simulink model "RobotArm"  (R2017b)
settings: Solver=FixedStepAuto  StartTime=0.0  StopTime=10  FixedStep=0.01  RelTol=1e-3
values from neighbouring files (symbols this model uses):
  K1 = 0.3415    [PDFUZZY.mat]    (also in gaPI_Fuzzy.m = par(bestchrom,1))
  K2 = 233.0301    [PDFUZZY.mat]    (also in gaPI_Fuzzy.m = par(bestchrom,2))
  K3 = 0.4831    [PDFUZZY.mat]    (also in gaPI_Fuzzy.m = par(bestchrom,3))
  K4 = 261.7584    [PDFUZZY.mat]    (also in gaPI_Fuzzy.m = par(bestchrom,4))
  Kd1 = par(bestchrom,3)-500    [GAthH.m]    (also in PIDVng.mat = 50.32; PIDsine.mat = 47.59; ga.m = par(bestchrom,3))
  Kd2 = par(bestchrom,6)-500    [GAthH.m]    (also in PIDVng.mat = 456.78; PIDsine.mat = 195.5; ga.m = par(bestchrom,6))
  Ki1 = par(bestchrom,2)-500    [GAthH.m]    (also in PIDVng.mat = 842.19; PIDsine.mat = 22.71; ga.m = par(bestchrom,2))
  Ki2 = par(bestchrom,5)-500    [GAthH.m]    (also in PIDVng.mat = 818.9; PIDsine.mat = 632.08; ga.m = par(bestchrom,5))
  Kp1 = par(bestchrom,1)-500    [GAthH.m]    (also in PIDVng.mat = 37.19; PIDsine.mat = 1.19; ga.m = par(bestchrom,1))
  Kp2 = par(bestchrom,4)-500    [GAthH.m]    (also in PIDVng.mat = 595.8; PIDsine.mat = 711.73; ga.m = par(bestchrom,4))
libraries: neural x50, fuzblock x2
(part 2 of 2)

== system RobotArm/PD_FUZZY_NEURAL /Custom Neural Network/Layer 2/LW{2,1} ==
  "ad{2,1}" : Inport  PortDimensions=20
      mask Display: e = 0.06;c1 = [120 230 180]/255;c2 = ([120 230 180]+0)/(256+128);c3 = ([120 230 180]+128)/(256+128);patch([0 1 1 0],[0 0 1 1],c1);patch([0 1 1 1-e 1-e 0+e],[0 0 1 1-e 0+e 0+e],c2);patch([0 0 1 1-e 0+e 0+e],[0 1 1 1-e 1-e 0+e],c3);plot([0 1 1 0 0],[0 0 1 1 0]);
  "IW{2,1}(1,:)'" : Constant  Value=[0.046554121912123817839113115724103408865630626678466796875;0.00016778847839335527133107495156849608974880538880825042724609375;0.01578686841424471742900692561306641437113285064697265625;-0.239614599437442177265467080360394902527332305908203125;-0.00822580942548027140015509672821281128562986850738525390625;-0.0333527887051501270576636670739389955997467041015625;0.006210181379244878070722268859071846236474812030792236328125;0.00900374076438229149765835046537176822312176227569580078125;-0.69848343780560673277335581587976776063442230224609375;-0.00280046923413862676455199363090287079103291034698486328125;0.004350649853579568841766000986126528005115687847137451171875;0.0662036547980797696055788037483580410480499267578125;0.004075788378211603855960643016942412941716611385345458984375;-0.64280666178294254553549080810626037418842315673828125;-0.0026488012173344521911488858023631109972484409809112548828125;-0.002129328380407683428410248183126896037720143795013427734375;-0.428133034077831264863078786220285110175609588623046875;0.129127304962275035737917505684890784323215484619140625;-0.006878772900469370087106479871863484731875360012054443359375;-0.0248842172997741743756261456610445748083293437957763671875]
      mask Display: e = 0.06;c1 = [120 150 230]/255;c2 = ([120 150 230]+0)/383;c3 = ([120 150 230]+128)/383;patch([0 1 1 0],[0 0 1 1],c1);patch([0 1 1 1-e 1-e 0+e],[0 0 1 1-e 0+e 0+e],c2);patch([0 0 1 1-e 0+e 0+e],[0 1 1 1-e 1-e 0+e],c3);plot([0 1 1 0 0],[0 0 1 1 0]);disp('weights');
  Mux : Mux  Inputs=1
      mask Display: e = 0.06;c1 = [120 150 230]/255;c2 = ([120 150 230]+0)/383;c3 = ([120 150 230]+128)/383;patch([0 1 1 0],[0 0 1 1],c1);patch([0 1 1 1-e 1-e 0+e],[0 0 1 1-e 0+e 0+e],c2);patch([0 0 1 1-e 0+e 0+e],[0 1 1 1-e 1-e 0+e],c3);plot([0 1 1 0 0],[0 0 1 1 0]);disp('Mux');
  dotprod1 : neural/Weight Functions/dotprod
      settings: SourceProductName=MATLAB Runtime - Deep Learning Toolbox  SourceProductBaseCode=Missing
  "lz{2,1}" : Outport
      mask Display: e = 0.06;c1 = [120 230 180]/255;c2 = ([120 230 180]+0)/(256+128);c3 = ([120 230 180]+128)/(256+128);patch([0 1 1 0],[0 0 1 1],c1);patch([0 1 1 1-e 1-e 0+e],[0 0 1 1-e 0+e 0+e],c2);patch([0 0 1 1-e 0+e 0+e],[0 1 1 1-e 1-e 0+e],c3);plot([0 1 1 0 0],[0 0 1 1 0]);
  wires:
  "IW{2,1}(1,:)'"/1 -> dotprod1/1
  "ad{2,1}"/1 -> dotprod1/2
  dotprod1/1 -> Mux/1
  Mux/1 -> "lz{2,1}"/1

== system RobotArm/PD_FUZZY_NEURAL /Custom Neural Network1/Layer 1/Delays 1 ==
  "p{1}" : Inport  PortDimensions=3
      mask Display: e = 0.06;c1 = [120 230 180]/255;c2 = ([120 230 180]+0)/(256+128);c3 = ([120 230 180]+128)/(256+128);patch([0 1 1 0],[0 0 1 1],c1);patch([0 1 1 1-e 1-e 0+e],[0 0 1 1-e 0+e 0+e],c2);patch([0 0 1 1-e 0+e 0+e],[0 1 1 1-e 1-e 0+e],c3);plot([0 1 1 0 0],[0 0 1 1 0]);
  mux : Mux  Inputs=1
      mask Display: e = 0.06;c1 = [120 150 230]/255;c2 = ([120 150 230]+0)/383;c3 = ([120 150 230]+128)/383;patch([0 1 1 0],[0 0 1 1],c1);patch([0 1 1 1-e 1-e 0+e],[0 0 1 1-e 0+e 0+e],c2);patch([0 0 1 1-e 0+e 0+e],[0 1 1 1-e 1-e 0+e],c3);plot([0 1 1 0 0],[0 0 1 1 0]);disp('Mux')
  "pd{1,1}" : Outport
      mask Display: e = 0.06;c1 = [120 230 180]/255;c2 = ([120 230 180]+0)/(256+128);c3 = ([120 230 180]+128)/(256+128);patch([0 1 1 0],[0 0 1 1],c1);patch([0 1 1 1-e 1-e 0+e],[0 0 1 1-e 0+e 0+e],c2);patch([0 0 1 1-e 0+e 0+e],[0 1 1 1-e 1-e 0+e],c3);plot([0 1 1 0 0],[0 0 1 1 0]);
  wires:
  "p{1}"/1 -> mux/1
  mux/1 -> "pd{1,1}"/1

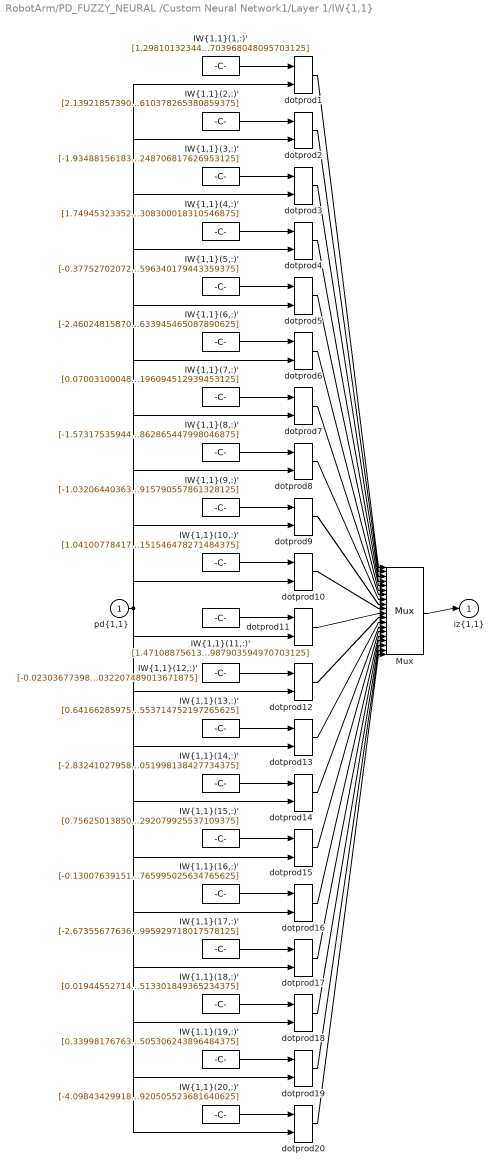
== system RobotArm/PD_FUZZY_NEURAL /Custom Neural Network1/Layer 1/IW{1,1} ==
  "pd{1,1}" : Inport  PortDimensions=3
      mask Display: e = 0.06;c1 = [120 230 180]/255;c2 = ([120 230 180]+0)/(256+128);c3 = ([120 230 180]+128)/(256+128);patch([0 1 1 0],[0 0 1 1],c1);patch([0 1 1 1-e 1-e 0+e],[0 0 1 1-e 0+e 0+e],c2);patch([0 0 1 1-e 0+e 0+e],[0 1 1 1-e 1-e 0+e],c3);plot([0 1 1 0 0],[0 0 1 1 0]);
  "IW{1,1}(1,:)'" : Constant  Value=[1.298101323448510147073875486967153847217559814453125;2.68668995949206479423310156562365591526031494140625;0.105680713798559811067434566211886703968048095703125]
      mask Display: e = 0.06;c1 = [120 150 230]/255;c2 = ([120 150 230]+0)/383;c3 = ([120 150 230]+128)/383;patch([0 1 1 0],[0 0 1 1],c1);patch([0 1 1 1-e 1-e 0+e],[0 0 1 1-e 0+e 0+e],c2);patch([0 0 1 1-e 0+e 0+e],[0 1 1 1-e 1-e 0+e],c3);plot([0 1 1 0 0],[0 0 1 1 0]);disp('Weights');
  "IW{1,1}(10,:)'" : Constant  Value=[1.041007784178143769082680591964162886142730712890625;1.0913679189835960858800945061375387012958526611328125;-3.79403971379421900422812541364692151546478271484375]
      mask Display: e = 0.06;c1 = [120 150 230]/255;c2 = ([120 150 230]+0)/383;c3 = ([120 150 230]+128)/383;patch([0 1 1 0],[0 0 1 1],c1);patch([0 1 1 1-e 1-e 0+e],[0 0 1 1-e 0+e 0+e],c2);patch([0 0 1 1-e 0+e 0+e],[0 1 1 1-e 1-e 0+e],c3);plot([0 1 1 0 0],[0 0 1 1 0]);disp('Weights');
  "IW{1,1}(11,:)'" : Constant  Value=[1.4710887561372587573060854992945678532123565673828125;-2.594021154299451126234998810105025768280029296875;-0.55809622186945173627492522427928633987903594970703125]
      mask Display: e = 0.06;c1 = [120 150 230]/255;c2 = ([120 150 230]+0)/383;c3 = ([120 150 230]+128)/383;patch([0 1 1 0],[0 0 1 1],c1);patch([0 1 1 1-e 1-e 0+e],[0 0 1 1-e 0+e 0+e],c2);patch([0 0 1 1-e 0+e 0+e],[0 1 1 1-e 1-e 0+e],c3);plot([0 1 1 0 0],[0 0 1 1 0]);disp('Weights');
  "IW{1,1}(12,:)'" : Constant  Value=[-0.02303677398099664153097165808503632433712482452392578125;-0.76517648256534098738512739146244712173938751220703125;0.019126199468667948178079996068845503032207489013671875]
      mask Display: e = 0.06;c1 = [120 150 230]/255;c2 = ([120 150 230]+0)/383;c3 = ([120 150 230]+128)/383;patch([0 1 1 0],[0 0 1 1],c1);patch([0 1 1 1-e 1-e 0+e],[0 0 1 1-e 0+e 0+e],c2);patch([0 0 1 1-e 0+e 0+e],[0 1 1 1-e 1-e 0+e],c3);plot([0 1 1 0 0],[0 0 1 1 0]);disp('Weights');
  "IW{1,1}(13,:)'" : Constant  Value=[0.641662859756776615682838382781483232975006103515625;1.648229245395270492480221946607343852519989013671875;3.25430695858256147090514787123538553714752197265625]
      mask Display: e = 0.06;c1 = [120 150 230]/255;c2 = ([120 150 230]+0)/383;c3 = ([120 150 230]+128)/383;patch([0 1 1 0],[0 0 1 1],c1);patch([0 1 1 1-e 1-e 0+e],[0 0 1 1-e 0+e 0+e],c2);patch([0 0 1 1-e 0+e 0+e],[0 1 1 1-e 1-e 0+e],c3);plot([0 1 1 0 0],[0 0 1 1 0]);disp('Weights');
  "IW{1,1}(14,:)'" : Constant  Value=[-2.83241027958725322122290890547446906566619873046875;-2.545638294362128295489355878089554607868194580078125;1.7885263091579071126346889286651276051998138427734375]
      mask Display: e = 0.06;c1 = [120 150 230]/255;c2 = ([120 150 230]+0)/383;c3 = ([120 150 230]+128)/383;patch([0 1 1 0],[0 0 1 1],c1);patch([0 1 1 1-e 1-e 0+e],[0 0 1 1-e 0+e 0+e],c2);patch([0 0 1 1-e 0+e 0+e],[0 1 1 1-e 1-e 0+e],c3);plot([0 1 1 0 0],[0 0 1 1 0]);disp('Weights');
  "IW{1,1}(15,:)'" : Constant  Value=[0.75625013850906885881641983360168524086475372314453125;2.0612501133497556082829760271124541759490966796875;3.430399247565897979939109063707292079925537109375]
      mask Display: e = 0.06;c1 = [120 150 230]/255;c2 = ([120 150 230]+0)/383;c3 = ([120 150 230]+128)/383;patch([0 1 1 0],[0 0 1 1],c1);patch([0 1 1 1-e 1-e 0+e],[0 0 1 1-e 0+e 0+e],c2);patch([0 0 1 1-e 0+e 0+e],[0 1 1 1-e 1-e 0+e],c3);plot([0 1 1 0 0],[0 0 1 1 0]);disp('Weights');
  "IW{1,1}(16,:)'" : Constant  Value=[-0.1300763915144957649783208353255758993327617645263671875;3.1475687752719210266150184907019138336181640625;-0.168673167062670492644116393421427346765995025634765625]
      mask Display: e = 0.06;c1 = [120 150 230]/255;c2 = ([120 150 230]+0)/383;c3 = ([120 150 230]+128)/383;patch([0 1 1 0],[0 0 1 1],c1);patch([0 1 1 1-e 1-e 0+e],[0 0 1 1-e 0+e 0+e],c2);patch([0 0 1 1-e 0+e 0+e],[0 1 1 1-e 1-e 0+e],c3);plot([0 1 1 0 0],[0 0 1 1 0]);disp('Weights');
  "IW{1,1}(17,:)'" : Constant  Value=[-2.673556776367207010736137817730195820331573486328125;-1.71981529092930518487492008716799318790435791015625;-0.450613133605147375693178446454112417995929718017578125]
      mask Display: e = 0.06;c1 = [120 150 230]/255;c2 = ([120 150 230]+0)/383;c3 = ([120 150 230]+128)/383;patch([0 1 1 0],[0 0 1 1],c1);patch([0 1 1 1-e 1-e 0+e],[0 0 1 1-e 0+e 0+e],c2);patch([0 0 1 1-e 0+e 0+e],[0 1 1 1-e 1-e 0+e],c3);plot([0 1 1 0 0],[0 0 1 1 0]);disp('Weights');
  "IW{1,1}(18,:)'" : Constant  Value=[0.019445527148039480624941433006824809126555919647216796875;0.9852408339296356842851309920661151409149169921875;0.02175143784294740478824081719722016714513301849365234375]
      mask Display: e = 0.06;c1 = [120 150 230]/255;c2 = ([120 150 230]+0)/383;c3 = ([120 150 230]+128)/383;patch([0 1 1 0],[0 0 1 1],c1);patch([0 1 1 1-e 1-e 0+e],[0 0 1 1-e 0+e 0+e],c2);patch([0 0 1 1-e 0+e 0+e],[0 1 1 1-e 1-e 0+e],c3);plot([0 1 1 0 0],[0 0 1 1 0]);disp('Weights');
  "IW{1,1}(19,:)'" : Constant  Value=[0.339981767632175746474132438379456289112567901611328125;-3.835244849837684544269222897128202021121978759765625;-1.3542732867112066141856985268532298505306243896484375]
      mask Display: e = 0.06;c1 = [120 150 230]/255;c2 = ([120 150 230]+0)/383;c3 = ([120 150 230]+128)/383;patch([0 1 1 0],[0 0 1 1],c1);patch([0 1 1 1-e 1-e 0+e],[0 0 1 1-e 0+e 0+e],c2);patch([0 0 1 1-e 0+e 0+e],[0 1 1 1-e 1-e 0+e],c3);plot([0 1 1 0 0],[0 0 1 1 0]);disp('Weights');
  "IW{1,1}(2,:)'" : Constant  Value=[2.1392185739000684208122038398869335651397705078125;1.281674728313323186057459679432213306427001953125;3.641787407070763205041430410346947610378265380859375]
      mask Display: e = 0.06;c1 = [120 150 230]/255;c2 = ([120 150 230]+0)/383;c3 = ([120 150 230]+128)/383;patch([0 1 1 0],[0 0 1 1],c1);patch([0 1 1 1-e 1-e 0+e],[0 0 1 1-e 0+e 0+e],c2);patch([0 0 1 1-e 0+e 0+e],[0 1 1 1-e 1-e 0+e],c3);plot([0 1 1 0 0],[0 0 1 1 0]);disp('Weights');
  "IW{1,1}(20,:)'" : Constant  Value=[-4.09843429918166979319948950433172285556793212890625;0.69057330462055477315885809730389155447483062744140625;0.0223408364389678683326057040403611608780920505523681640625]
      mask Display: e = 0.06;c1 = [120 150 230]/255;c2 = ([120 150 230]+0)/383;c3 = ([120 150 230]+128)/383;patch([0 1 1 0],[0 0 1 1],c1);patch([0 1 1 1-e 1-e 0+e],[0 0 1 1-e 0+e 0+e],c2);patch([0 0 1 1-e 0+e 0+e],[0 1 1 1-e 1-e 0+e],c3);plot([0 1 1 0 0],[0 0 1 1 0]);disp('Weights');
  "IW{1,1}(3,:)'" : Constant  Value=[-1.93488156183017512290689410292543470859527587890625;2.103172833789326734432734156143851578235626220703125;-2.540487994611002608991157103446312248706817626953125]
      mask Display: e = 0.06;c1 = [120 150 230]/255;c2 = ([120 150 230]+0)/383;c3 = ([120 150 230]+128)/383;patch([0 1 1 0],[0 0 1 1],c1);patch([0 1 1 1-e 1-e 0+e],[0 0 1 1-e 0+e 0+e],c2);patch([0 0 1 1-e 0+e 0+e],[0 1 1 1-e 1-e 0+e],c3);plot([0 1 1 0 0],[0 0 1 1 0]);disp('Weights');
  "IW{1,1}(4,:)'" : Constant  Value=[1.7494532335268075939893606118857860565185546875;3.050495676388021326630450857919640839099884033203125;-0.92830260598007707795176202125730924308300018310546875]
      mask Display: e = 0.06;c1 = [120 150 230]/255;c2 = ([120 150 230]+0)/383;c3 = ([120 150 230]+128)/383;patch([0 1 1 0],[0 0 1 1],c1);patch([0 1 1 1-e 1-e 0+e],[0 0 1 1-e 0+e 0+e],c2);patch([0 0 1 1-e 0+e 0+e],[0 1 1 1-e 1-e 0+e],c3);plot([0 1 1 0 0],[0 0 1 1 0]);disp('Weights');
  "IW{1,1}(5,:)'" : Constant  Value=[-0.37752702072625432538899303835933096706867218017578125;-1.137271367403070332358083760482259094715118408203125;1.551047187862562903859497964731417596340179443359375]
      mask Display: e = 0.06;c1 = [120 150 230]/255;c2 = ([120 150 230]+0)/383;c3 = ([120 150 230]+128)/383;patch([0 1 1 0],[0 0 1 1],c1);patch([0 1 1 1-e 1-e 0+e],[0 0 1 1-e 0+e 0+e],c2);patch([0 0 1 1-e 0+e 0+e],[0 1 1 1-e 1-e 0+e],c3);plot([0 1 1 0 0],[0 0 1 1 0]);disp('Weights');
  "IW{1,1}(6,:)'" : Constant  Value=[-2.460248158700125031828065402805805206298828125;0.84061468188021704062151684411219321191310882568359375;2.31296954212943006723435246385633945465087890625]
      mask Display: e = 0.06;c1 = [120 150 230]/255;c2 = ([120 150 230]+0)/383;c3 = ([120 150 230]+128)/383;patch([0 1 1 0],[0 0 1 1],c1);patch([0 1 1 1-e 1-e 0+e],[0 0 1 1-e 0+e 0+e],c2);patch([0 0 1 1-e 0+e 0+e],[0 1 1 1-e 1-e 0+e],c3);plot([0 1 1 0 0],[0 0 1 1 0]);disp('Weights');
  "IW{1,1}(7,:)'" : Constant  Value=[0.0700310004863720914070057688149972818791866302490234375;-1.6712400212012938904848624588339589536190032958984375;-0.0815120027134079994102222599394735880196094512939453125]
      mask Display: e = 0.06;c1 = [120 150 230]/255;c2 = ([120 150 230]+0)/383;c3 = ([120 150 230]+128)/383;patch([0 1 1 0],[0 0 1 1],c1);patch([0 1 1 1-e 1-e 0+e],[0 0 1 1-e 0+e 0+e],c2);patch([0 0 1 1-e 0+e 0+e],[0 1 1 1-e 1-e 0+e],c3);plot([0 1 1 0 0],[0 0 1 1 0]);disp('Weights');
  "IW{1,1}(8,:)'" : Constant  Value=[-1.5731753594485500258315369137562811374664306640625;-1.1714016532727262731583550703362561762332916259765625;3.363686937816534605616425324114970862865447998046875]
      mask Display: e = 0.06;c1 = [120 150 230]/255;c2 = ([120 150 230]+0)/383;c3 = ([120 150 230]+128)/383;patch([0 1 1 0],[0 0 1 1],c1);patch([0 1 1 1-e 1-e 0+e],[0 0 1 1-e 0+e 0+e],c2);patch([0 0 1 1-e 0+e 0+e],[0 1 1 1-e 1-e 0+e],c3);plot([0 1 1 0 0],[0 0 1 1 0]);disp('Weights');
  "IW{1,1}(9,:)'" : Constant  Value=[-1.0320644036352526473621082914178259670734405517578125;-1.4924801652789827510758868811535649001598358154296875;-0.71115224162992252132653447915799915790557861328125]
      mask Display: e = 0.06;c1 = [120 150 230]/255;c2 = ([120 150 230]+0)/383;c3 = ([120 150 230]+128)/383;patch([0 1 1 0],[0 0 1 1],c1);patch([0 1 1 1-e 1-e 0+e],[0 0 1 1-e 0+e 0+e],c2);patch([0 0 1 1-e 0+e 0+e],[0 1 1 1-e 1-e 0+e],c3);plot([0 1 1 0 0],[0 0 1 1 0]);disp('Weights');
  Mux : Mux  Inputs=20
      mask Display: e = 0.06;c1 = [120 150 230]/255;c2 = ([120 150 230]+0)/383;c3 = ([120 150 230]+128)/383;patch([0 1 1 0],[0 0 1 1],c1);patch([0 1 1 1-e 1-e 0+e],[0 0 1 1-e 0+e 0+e],c2);patch([0 0 1 1-e 0+e 0+e],[0 1 1 1-e 1-e 0+e],c3);plot([0 1 1 0 0],[0 0 1 1 0]);disp('Mux');
  dotprod{1..20} (20 alike) : neural/Weight Functions/dotprod
      settings: SourceProductName=MATLAB Runtime - Deep Learning Toolbox  SourceProductBaseCode=Missing
  "iz{1,1}" : Outport
      mask Display: e = 0.06;c1 = [120 230 180]/255;c2 = ([120 230 180]+0)/(256+128);c3 = ([120 230 180]+128)/(256+128);patch([0 1 1 0],[0 0 1 1],c1);patch([0 1 1 1-e 1-e 0+e],[0 0 1 1-e 0+e 0+e],c2);patch([0 0 1 1-e 0+e 0+e],[0 1 1 1-e 1-e 0+e],c3);plot([0 1 1 0 0],[0 0 1 1 0]);
  wires:
  "IW{1,1}(1,:)'"/1 -> dotprod1/1
  "pd{1,1}"/1 -> dotprod1/2, dotprod2/2, dotprod3/2, dotprod4/2, dotprod5/2, dotprod6/2, dotprod7/2, dotprod8/2, dotprod9/2, dotprod10/2, dotprod11/2, dotprod12/2, dotprod13/2, dotprod14/2, dotprod15/2, dotprod16/2, dotprod17/2, dotprod18/2, dotprod19/2, dotprod20/2
  dotprod1/1 -> Mux/1
  "IW{1,1}(2,:)'"/1 -> dotprod2/1
  dotprod2/1 -> Mux/2
  "IW{1,1}(3,:)'"/1 -> dotprod3/1
  dotprod3/1 -> Mux/3
  "IW{1,1}(4,:)'"/1 -> dotprod4/1
  dotprod4/1 -> Mux/4
  "IW{1,1}(5,:)'"/1 -> dotprod5/1
  dotprod5/1 -> Mux/5
  "IW{1,1}(6,:)'"/1 -> dotprod6/1
  dotprod6/1 -> Mux/6
  "IW{1,1}(7,:)'"/1 -> dotprod7/1
  dotprod7/1 -> Mux/7
  "IW{1,1}(8,:)'"/1 -> dotprod8/1
  dotprod8/1 -> Mux/8
  "IW{1,1}(9,:)'"/1 -> dotprod9/1
  dotprod9/1 -> Mux/9
  "IW{1,1}(10,:)'"/1 -> dotprod10/1
  dotprod10/1 -> Mux/10
  "IW{1,1}(11,:)'"/1 -> dotprod11/1
  dotprod11/1 -> Mux/11
  "IW{1,1}(12,:)'"/1 -> dotprod12/1
  dotprod12/1 -> Mux/12
  "IW{1,1}(13,:)'"/1 -> dotprod13/1
  dotprod13/1 -> Mux/13
  "IW{1,1}(14,:)'"/1 -> dotprod14/1
  dotprod14/1 -> Mux/14
  "IW{1,1}(15,:)'"/1 -> dotprod15/1
  dotprod15/1 -> Mux/15
  "IW{1,1}(16,:)'"/1 -> dotprod16/1
  dotprod16/1 -> Mux/16
  "IW{1,1}(17,:)'"/1 -> dotprod17/1
  dotprod17/1 -> Mux/17
  "IW{1,1}(18,:)'"/1 -> dotprod18/1
  dotprod18/1 -> Mux/18
  "IW{1,1}(19,:)'"/1 -> dotprod19/1
  dotprod19/1 -> Mux/19
  "IW{1,1}(20,:)'"/1 -> dotprod20/1
  dotprod20/1 -> Mux/20
  Mux/1 -> "iz{1,1}"/1

== system RobotArm/PD_FUZZY_NEURAL /Custom Neural Network1/Layer 2/Delays 1 ==
  "p{2}" : Inport  PortDimensions=20
      mask Display: e = 0.06;c1 = [120 230 180]/255;c2 = ([120 230 180]+0)/(256+128);c3 = ([120 230 180]+128)/(256+128);patch([0 1 1 0],[0 0 1 1],c1);patch([0 1 1 1-e 1-e 0+e],[0 0 1 1-e 0+e 0+e],c2);patch([0 0 1 1-e 0+e 0+e],[0 1 1 1-e 1-e 0+e],c3);plot([0 1 1 0 0],[0 0 1 1 0]);
  mux : Mux  Inputs=1
      mask Display: e = 0.06;c1 = [120 150 230]/255;c2 = ([120 150 230]+0)/383;c3 = ([120 150 230]+128)/383;patch([0 1 1 0],[0 0 1 1],c1);patch([0 1 1 1-e 1-e 0+e],[0 0 1 1-e 0+e 0+e],c2);patch([0 0 1 1-e 0+e 0+e],[0 1 1 1-e 1-e 0+e],c3);plot([0 1 1 0 0],[0 0 1 1 0]);disp('Mux')
  "pd{2,1}" : Outport
      mask Display: e = 0.06;c1 = [120 230 180]/255;c2 = ([120 230 180]+0)/(256+128);c3 = ([120 230 180]+128)/(256+128);patch([0 1 1 0],[0 0 1 1],c1);patch([0 1 1 1-e 1-e 0+e],[0 0 1 1-e 0+e 0+e],c2);patch([0 0 1 1-e 0+e 0+e],[0 1 1 1-e 1-e 0+e],c3);plot([0 1 1 0 0],[0 0 1 1 0]);
  wires:
  "p{2}"/1 -> mux/1
  mux/1 -> "pd{2,1}"/1

== system RobotArm/PD_FUZZY_NEURAL /Custom Neural Network1/Layer 2/LW{2,1} ==
  "ad{2,1}" : Inport  PortDimensions=20
      mask Display: e = 0.06;c1 = [120 230 180]/255;c2 = ([120 230 180]+0)/(256+128);c3 = ([120 230 180]+128)/(256+128);patch([0 1 1 0],[0 0 1 1],c1);patch([0 1 1 1-e 1-e 0+e],[0 0 1 1-e 0+e 0+e],c2);patch([0 0 1 1-e 0+e 0+e],[0 1 1 1-e 1-e 0+e],c3);plot([0 1 1 0 0],[0 0 1 1 0]);
  "IW{2,1}(1,:)'" : Constant  Value=[0.0260805455288128616719856012196032679639756679534912109375;-0.0031325125071500238560506801377414376474916934967041015625;0.000495277192721998754838808043388098667492158710956573486328125;0.00760022526004941294253125505520074511878192424774169921875;-0.0263516857164060348817091750106555991806089878082275390625;-0.0016089836069958919455291646016803497332148253917694091796875;-0.2184122450427620487634072787841432727873325347900390625;-0.0029588715963936198898032170490068892831914126873016357421875;-0.0273822407903332697143294893749043694697320461273193359375;0.004138516217546377683189628982063368312083184719085693359375;-0.003159027568638029907777120541823023813776671886444091796875;-0.9902167581888929870359561391524039208889007568359375;0.0037499174366412576196727624022742020315490663051605224609375;0.000113241343670208036912942783924762579772504977881908416748046875;-0.00080791394197934581801467945894046351895667612552642822265625;0.09905169767753442544577779926839866675436496734619140625;-0.0032117176773793104128940090191690615029074251651763916015625;0.49141222259313799280988632744993083178997039794921875;-0.05196827081355660793438033806523890234529972076416015625;-0.0030436726907445456336009925735197612084448337554931640625]
      mask Display: e = 0.06;c1 = [120 150 230]/255;c2 = ([120 150 230]+0)/383;c3 = ([120 150 230]+128)/383;patch([0 1 1 0],[0 0 1 1],c1);patch([0 1 1 1-e 1-e 0+e],[0 0 1 1-e 0+e 0+e],c2);patch([0 0 1 1-e 0+e 0+e],[0 1 1 1-e 1-e 0+e],c3);plot([0 1 1 0 0],[0 0 1 1 0]);disp('weights');
  Mux : Mux  Inputs=1
      mask Display: e = 0.06;c1 = [120 150 230]/255;c2 = ([120 150 230]+0)/383;c3 = ([120 150 230]+128)/383;patch([0 1 1 0],[0 0 1 1],c1);patch([0 1 1 1-e 1-e 0+e],[0 0 1 1-e 0+e 0+e],c2);patch([0 0 1 1-e 0+e 0+e],[0 1 1 1-e 1-e 0+e],c3);plot([0 1 1 0 0],[0 0 1 1 0]);disp('Mux');
  dotprod1 : neural/Weight Functions/dotprod
      settings: SourceProductName=MATLAB Runtime - Deep Learning Toolbox  SourceProductBaseCode=Missing
  "lz{2,1}" : Outport
      mask Display: e = 0.06;c1 = [120 230 180]/255;c2 = ([120 230 180]+0)/(256+128);c3 = ([120 230 180]+128)/(256+128);patch([0 1 1 0],[0 0 1 1],c1);patch([0 1 1 1-e 1-e 0+e],[0 0 1 1-e 0+e 0+e],c2);patch([0 0 1 1-e 0+e 0+e],[0 1 1 1-e 1-e 0+e],c3);plot([0 1 1 0 0],[0 0 1 1 0]);
  wires:
  "IW{2,1}(1,:)'"/1 -> dotprod1/1
  "ad{2,1}"/1 -> dotprod1/2
  dotprod1/1 -> Mux/1
  Mux/1 -> "lz{2,1}"/1

== matlab function RobotArm/2DOF/MATLAB Function ==
  data: the input; M_inv output; the_dot input; V output; G output
function [M_inv, V, G] = fcn(the, the_dot)
the1 = the(1); the2 = the(2); the1_dot = the_dot(1); the2_dot = the_dot(2);
s2 = sin(the2); c2 = cos(the2); c12 = cos(the1+the2);
c1= cos(the1);   

g = 9.8;
l1 = 0.6; l2 = 0.4; m2 = 1; m1 = 1;
g1 =  m2*l2*g*c12 + (m1+m2)*l1*g*c1;
g2 = m2*l2*g*c12;

v1 = - m2*l1*l2*s2*the2_dot*the2_dot - 2*m2*l1*l2*s2*the1_dot*the2_dot;
v2 =   m2*l1*l2*s2*the1_dot*the1_dot;

M11 = m2*l2*l2 + 2*l1*l2*m2*c2 + l1*l1*(m1+m2);
M12 = m2*l2*l2 + l1*l2*m2*c2 ;
M21 = m2*l2*l2 + l1*l2*m2*c2 ;
M22 = m1*l2*l2 ;

V = [v1;v2]; G = [g1;g2];
M_inv = inv([M11 M12; M21 M22]);

== matlab function RobotArm/2DOF3/MATLAB Function ==
  data: the input; M_inv output; the_dot input; V output; G output
function [M_inv, V, G] = fcn(the, the_dot)
the1 = the(1); the2 = the(2); the1_dot = the_dot(1); the2_dot = the_dot(2);
s2 = sin(the2); c2 = cos(the2); c12 = cos(the1+the2);
c1= cos(the1);   

g = 9.8;
l1 = 0.6; l2 = 0.4; m2 = 1; m1 = 1;
g1 =  m2*l2*g*c12 + (m1+m2)*l1*g*c1;
g2 = m2*l2*g*c12;

v1 = - m2*l1*l2*s2*the2_dot*the2_dot - 2*m2*l1*l2*s2*the1_dot*the2_dot;
v2 =   m2*l1*l2*s2*the1_dot*the1_dot;

M11 = m2*l2*l2 + 2*l1*l2*m2*c2 + l1*l1*(m1+m2);
M12 = m2*l2*l2 + l1*l2*m2*c2 ;
M21 = m2*l2*l2 + l1*l2*m2*c2 ;
M22 = m1*l2*l2 ;

V = [v1;v2]; G = [g1;g2];
M_inv = inv([M11 M12; M21 M22]);

== matlab function RobotArm/2DOF2/MATLAB Function ==
  data: the input; M_inv output; the_dot input; V output; G output
function [M_inv, V, G] = fcn(the, the_dot)
the1 = the(1); the2 = the(2); the1_dot = the_dot(1); the2_dot = the_dot(2);
s2 = sin(the2); c2 = cos(the2); c12 = cos(the1+the2);
c1= cos(the1);   

g = 9.8;
l1 = 0.6; l2 = 0.4; m2 = 1; m1 = 1;
g1 =  m2*l2*g*c12 + (m1+m2)*l1*g*c1;
g2 = m2*l2*g*c12;

v1 = - m2*l1*l2*s2*the2_dot*the2_dot - 2*m2*l1*l2*s2*the1_dot*the2_dot;
v2 =   m2*l1*l2*s2*the1_dot*the1_dot;

M11 = m2*l2*l2 + 2*l1*l2*m2*c2 + l1*l1*(m1+m2);
M12 = m2*l2*l2 + l1*l2*m2*c2 ;
M21 = m2*l2*l2 + l1*l2*m2*c2 ;
M22 = m1*l2*l2 ;

V = [v1;v2]; G = [g1;g2];
M_inv = inv([M11 M12; M21 M22]);

== matlab function RobotArm/MATLAB Function ==
  data: theta input; y output
function y = checkJoint1(theta)
if (theta>2*pi)
    y=1;
    disp('JOINT 1 ERROR: Angle of joint 1 more than 360 degree!');
elseif (theta<-2*pi)
    y=1;
    disp('JOINT 1 ERROR: Angle of joint 1 less than -360 degree!');
else
    y=0;
end

== matlab function RobotArm/MATLAB Function1 ==
  data: theta input; y output
function y = checkJoint2(theta)
if (theta>2*pi)
    y=1;
    disp('JOINT 2 ERROR: Angle of joint 2 more than 360 degree!');
elseif (theta<-2*pi)
    y=1;
    disp('JOINT 2 ERROR: Angle of joint 2 less than -360 degree!');
else
    y=0;
end
